simulink model "stepper_motor_driver_model"  (R2012b)
settings: Solver=ode45  StartTime=0.0  StopTime=10.0  RelTol=1e-3
libraries: elec_lib x21, fl_lib x10, nesl_utility x6
settings Model: Creator=Computer  LastModifiedBy=Computer

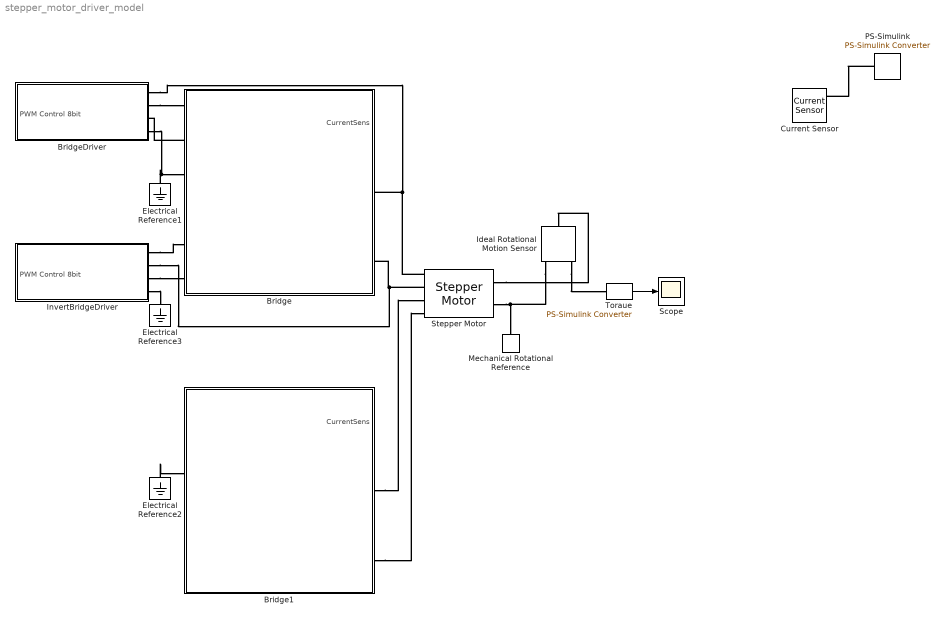
== system stepper_motor_driver_model ==
  Bridge : Subsystem
  Bridge1 : Subsystem
  BridgeDriver : Subsystem
  Current Sensor : fl_lib/Electrical/Electrical Sensors/Current Sensor  i1_Log=off  v1_Log=off  LocalVarNames=|i1|v1  LocalVarDescs=|i1|v1  LocalVarLogging=[0 0]
  Electrical Reference1 : fl_lib/Electrical/Electrical Elements/Electrical Reference  i_Log=off  LocalVarNames=|v1  LocalVarDescs=|v1  LocalVarLogging=[]
  Electrical Reference2 : fl_lib/Electrical/Electrical Elements/Electrical Reference  i_Log=off  LocalVarNames=|v1  LocalVarDescs=|v1  LocalVarLogging=[]
  Electrical Reference3 : fl_lib/Electrical/Electrical Elements/Electrical Reference  i_Log=off  LocalVarNames=|v1  LocalVarDescs=|v1  LocalVarLogging=[]
  Ideal Rotational Motion Sensor : fl_lib/Mechanical/Mechanical Sensors/Ideal Rotational Motion Sensor  offset=0 rad  w_Log=off  t_Log=off  phi_Log=off  LocalVarNames=|w|t|phi  LocalVarDescs=|w|t|phi  LocalVarLogging=[]
  InvertBridgeDriver : Subsystem
  Mechanical Rotational Reference : fl_lib/Mechanical/Rotational Elements/Mechanical Rotational Reference  t_Log=off  LocalVarNames=|t  LocalVarDescs=|t  LocalVarLogging=0
  PS-Simulink : nesl_utility/PS-Simulink Converter  PhysicalDomain=network_engine_domain  LeftPortType=input  RightPortType=output  SubClassName=ps_output  PseudoPeriodic=off  Frequencies=[]  Unit=A  AffineConversion=off
  Scope : Scope
  Stepper Motor : elec_lib/Actuators & Drivers/Rotational Actuators/Stepper Motor  Ra=0.55 Ohm  La=0.0015 H  Km=0.19 N*m/A  Rm=Inf Ohm  Step=1.8 deg  J=4.5e-5 kg*m^2  B=8e-4 N*m/(rad/s)  speed0=0 rpm  theta0=0 deg  LocalVarLogging=[]  alpha=[ 0.00393 0.00393 ] 1/K  Tmeas=25 C  thermal_masses=[ 100 100 ] J/K  initial_temperatures=[ 25 25 ] C  rotor_thermal_mass=50 J/K  rotor_initial_temperature=25 C  Rm_percent_rotor=90
  "Toraue " : nesl_utility/PS-Simulink Converter  PhysicalDomain=network_engine_domain  LeftPortType=input  RightPortType=output  SubClassName=ps_output  PseudoPeriodic=off  Frequencies=[]  Unit=N*m  AffineConversion=off
  wires:
  "Toraue "/1 -> Scope/1
  connections:
  Stepper Motor/RConn2 -- Ideal Rotational Motion Sensor/RConn1 -- Mechanical Rotational Reference/LConn1
  Ideal Rotational Motion Sensor/RConn3 -- "Toraue "/LConn1
  Stepper Motor/RConn1 -- Ideal Rotational Motion Sensor/LConn1
  PS-Simulink/LConn1 -- Current Sensor/RConn1
  Stepper Motor/LConn2 -- InvertBridgeDriver/RConn2 -- Bridge/RConn2
  Stepper Motor/LConn1 -- BridgeDriver/RConn1 -- Bridge/RConn1
  Bridge1/RConn1 -- Stepper Motor/LConn3
  Bridge1/RConn2 -- Stepper Motor/LConn4
  Electrical Reference1/LConn1 -- BridgeDriver/RConn4 -- Bridge/LConn3
  Electrical Reference2/LConn1 -- Bridge1/LConn3
  Bridge/LConn2 -- BridgeDriver/RConn3
  BridgeDriver/RConn2 -- Bridge/LConn1
  InvertBridgeDriver/RConn4 -- Electrical Reference3/LConn1
  InvertBridgeDriver/RConn3 -- Bridge/LConn6
  InvertBridgeDriver/RConn1 -- Bridge/LConn5

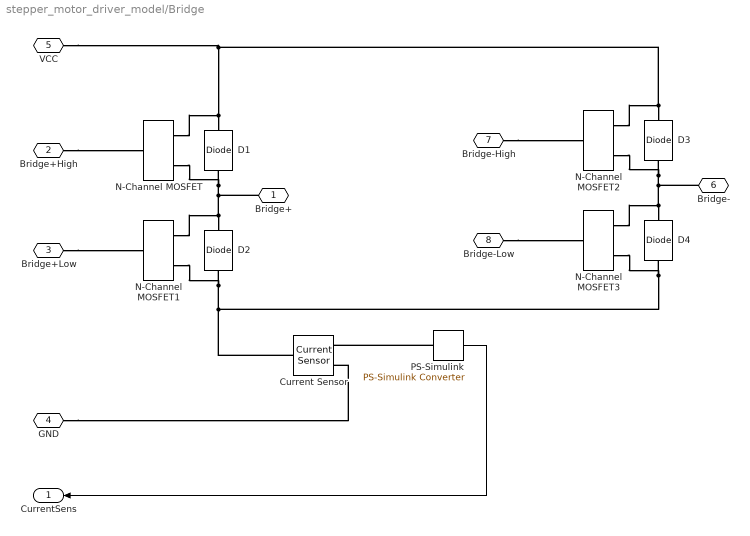
== system stepper_motor_driver_model/Bridge ==
  Current Sensor : fl_lib/Electrical/Electrical Sensors/Current Sensor  i1_Log=off  v1_Log=off  LocalVarNames=|i1|v1  LocalVarDescs=|i1|v1  LocalVarLogging=[0 0]
  D{1..4} (4 alike) : elec_lib/Semiconductor Devices/Diode  ModelType=3  Vf=0.6 V  Ron=0.3 Ohm  Goff=1e-8 S  Rz=0.3 Ohm  Vz=50 V  C_PWL=5 pF  prmExp=1  I12=[ 0.25 5 ] A  V12=[ 0.7 0.8 ] V  I1=0.07 A  V1=0.7 V  RS=0.01 Ohm  IS=1e-14 A  Tmeas=25 C  ec=1  BV=Inf V  C_param=1  CJ0=100 pF  VJ=1 V  Mgrad=0.5  Vvec=[ 0.1 10 100 ] V  Cvec=[ 3.5 1 0.4 ] pF  FC=0.5  Q_param=1  Irrm=-7.15 A  iF=4 A  didt=-750 A/us  trr=115 ns  TT=50 ns  tau=100 ns  T_param=1  IS_T2=1.25e-7 A  I1_T2=0.245 A  V1_T2=0.5 V  Tmeas2=125 C  EG_param=1  EG=1.11 eV  XTI_param=1  XTI=3  dBVdT=0 V/K  Tdevice=25 C  LocalVarLogging=[]  Rth=[ 0 10 ] K/W  thermal_mass_parameterization=1  thermal_mass=[ 0 1 ] J/K  thermal_time_constant=[ 0 10 ] s  thermal_mass_initial_temperatures=[ 25 25 ] C
  N-Channel MOSFET{,1..3} (4 alike) : elec_lib/Semiconductor Devices/N-Channel MOSFET  parameterization=1  prmDatasheet=1  prmEquCoeff=1  Beta=5 A/V^2  Rds=0.025 Ohm  Id=6 A  Vgs=10 V  Vth=1.7 V  lam=0 1/V  Tmeas=25 C  RS=1e-4 Ohm  RD=0.01 Ohm  C_param=1  C_GS=270 pF  C_GD=80 pF  C_iss=350 pF  C_rss=80 pF  dVth_dT=-6 mV/K  Rds_T2=0.037 Ohm  Tmeas2=125 C  BEXDatasheet=-1.5  BEXEquCoeff=-1.5  TdeviceDatasheet=25 C  TdeviceEquCoeff=25 C  LocalVarLogging=[]  Rth=[ 0 10 ] K/W  thermal_mass_parameterization=1  thermal_mass=[ 0 1 ] J/K  thermal_time_constant=[ 0 10 ] s  thermal_mass_initial_temperatures=[ 25 25 ] C
  PS-Simulink : nesl_utility/PS-Simulink Converter  PhysicalDomain=network_engine_domain  LeftPortType=input  RightPortType=output  SubClassName=ps_output  PseudoPeriodic=off  Frequencies=[]  Unit=A  AffineConversion=off
  Bridge+ : PMIOPort  Port=1  Side=Right
  Bridge+High : PMIOPort  Port=2  Side=Left
  Bridge+Low : PMIOPort  Port=3  Side=Left
  "GND " : PMIOPort  Port=4  Side=Left
  VCC : PMIOPort  Port=5  Side=Left
  Bridge- : PMIOPort  Port=6  Side=Right
  Bridge-High : PMIOPort  Port=7  Side=Left
  Bridge-Low : PMIOPort  Port=8  Side=Left
  CurrentSens : Outport
  wires:
  PS-Simulink/1 -> CurrentSens/1
  connections:
  N-Channel MOSFET1/RConn1 -- Bridge+/RConn1 -- N-Channel MOSFET/RConn2 -- D1/LConn1 -- D2/RConn1
  D4/LConn1 -- N-Channel MOSFET1/RConn2 -- D2/LConn1 -- Current Sensor/LConn1 -- N-Channel MOSFET3/RConn2
  N-Channel MOSFET2/RConn1 -- D1/RConn1 -- N-Channel MOSFET/RConn1 -- VCC/RConn1 -- D3/RConn1
  Bridge+High/RConn1 -- N-Channel MOSFET/LConn1
  Bridge+Low/RConn1 -- N-Channel MOSFET1/LConn1
  PS-Simulink/LConn1 -- Current Sensor/RConn1
  "GND "/RConn1 -- Current Sensor/RConn2
  N-Channel MOSFET3/RConn1 -- Bridge-/RConn1 -- N-Channel MOSFET2/RConn2 -- D3/LConn1 -- D4/RConn1
  Bridge-High/RConn1 -- N-Channel MOSFET2/LConn1
  Bridge-Low/RConn1 -- N-Channel MOSFET3/LConn1

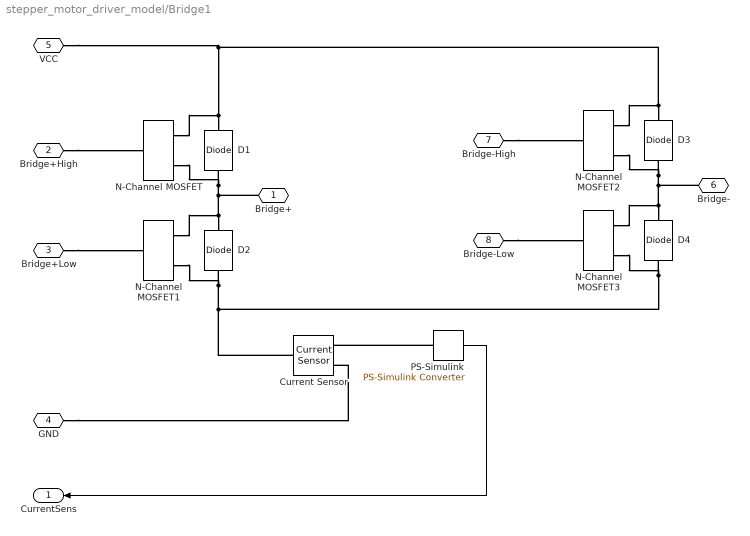
== system stepper_motor_driver_model/Bridge1 ==
  Current Sensor : fl_lib/Electrical/Electrical Sensors/Current Sensor  i1_Log=off  v1_Log=off  LocalVarNames=|i1|v1  LocalVarDescs=|i1|v1  LocalVarLogging=[0 0]
  D{1..4} (4 alike) : elec_lib/Semiconductor Devices/Diode  ModelType=3  Vf=0.6 V  Ron=0.3 Ohm  Goff=1e-8 S  Rz=0.3 Ohm  Vz=50 V  C_PWL=5 pF  prmExp=1  I12=[ 0.25 5 ] A  V12=[ 0.7 0.8 ] V  I1=0.07 A  V1=0.7 V  RS=0.01 Ohm  IS=1e-14 A  Tmeas=25 C  ec=1  BV=Inf V  C_param=1  CJ0=100 pF  VJ=1 V  Mgrad=0.5  Vvec=[ 0.1 10 100 ] V  Cvec=[ 3.5 1 0.4 ] pF  FC=0.5  Q_param=1  Irrm=-7.15 A  iF=4 A  didt=-750 A/us  trr=115 ns  TT=50 ns  tau=100 ns  T_param=1  IS_T2=1.25e-7 A  I1_T2=0.245 A  V1_T2=0.5 V  Tmeas2=125 C  EG_param=1  EG=1.11 eV  XTI_param=1  XTI=3  dBVdT=0 V/K  Tdevice=25 C  LocalVarLogging=[]  Rth=[ 0 10 ] K/W  thermal_mass_parameterization=1  thermal_mass=[ 0 1 ] J/K  thermal_time_constant=[ 0 10 ] s  thermal_mass_initial_temperatures=[ 25 25 ] C
  N-Channel MOSFET{,1..3} (4 alike) : elec_lib/Semiconductor Devices/N-Channel MOSFET  parameterization=1  prmDatasheet=1  prmEquCoeff=1  Beta=5 A/V^2  Rds=0.025 Ohm  Id=6 A  Vgs=10 V  Vth=1.7 V  lam=0 1/V  Tmeas=25 C  RS=1e-4 Ohm  RD=0.01 Ohm  C_param=1  C_GS=270 pF  C_GD=80 pF  C_iss=350 pF  C_rss=80 pF  dVth_dT=-6 mV/K  Rds_T2=0.037 Ohm  Tmeas2=125 C  BEXDatasheet=-1.5  BEXEquCoeff=-1.5  TdeviceDatasheet=25 C  TdeviceEquCoeff=25 C  LocalVarLogging=[]  Rth=[ 0 10 ] K/W  thermal_mass_parameterization=1  thermal_mass=[ 0 1 ] J/K  thermal_time_constant=[ 0 10 ] s  thermal_mass_initial_temperatures=[ 25 25 ] C
  PS-Simulink : nesl_utility/PS-Simulink Converter  PhysicalDomain=network_engine_domain  LeftPortType=input  RightPortType=output  SubClassName=ps_output  PseudoPeriodic=off  Frequencies=[]  Unit=A  AffineConversion=off
  Bridge+ : PMIOPort  Port=1  Side=Right
  Bridge+High : PMIOPort  Port=2  Side=Left
  Bridge+Low : PMIOPort  Port=3  Side=Left
  "GND " : PMIOPort  Port=4  Side=Left
  VCC : PMIOPort  Port=5  Side=Left
  Bridge- : PMIOPort  Port=6  Side=Right
  Bridge-High : PMIOPort  Port=7  Side=Left
  Bridge-Low : PMIOPort  Port=8  Side=Left
  CurrentSens : Outport
  wires:
  PS-Simulink/1 -> CurrentSens/1
  connections:
  N-Channel MOSFET/RConn2 -- D1/LConn1 -- D2/RConn1 -- N-Channel MOSFET1/RConn1 -- Bridge+/RConn1
  N-Channel MOSFET1/RConn2 -- D2/LConn1 -- Current Sensor/LConn1 -- N-Channel MOSFET3/RConn2 -- D4/LConn1
  D1/RConn1 -- N-Channel MOSFET/RConn1 -- VCC/RConn1 -- D3/RConn1 -- N-Channel MOSFET2/RConn1
  Bridge+High/RConn1 -- N-Channel MOSFET/LConn1
  Bridge+Low/RConn1 -- N-Channel MOSFET1/LConn1
  PS-Simulink/LConn1 -- Current Sensor/RConn1
  "GND "/RConn1 -- Current Sensor/RConn2
  Bridge-/RConn1 -- N-Channel MOSFET2/RConn2 -- D3/LConn1 -- D4/RConn1 -- N-Channel MOSFET3/RConn1
  Bridge-High/RConn1 -- N-Channel MOSFET2/LConn1
  Bridge-Low/RConn1 -- N-Channel MOSFET3/LConn1

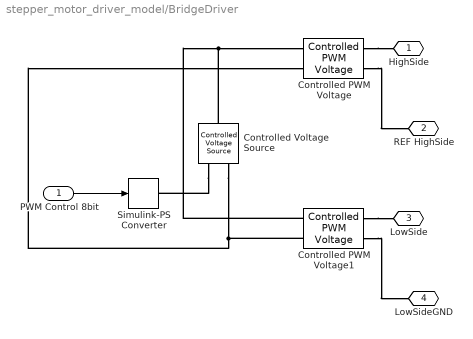
== system stepper_motor_driver_model/BridgeDriver ==
  PWM Control 8bit : Inport
  Controlled PWM Voltage : elec_lib/Actuators & Drivers/Drivers/Controlled PWM Voltage  F=150 kHz  TD=0 s  pulse_width_offset=0 s  Vmin=0 V  Vmax=255 V  Vm=10 V  pwm_or_av=1  event_type=1  sample_time=1e-6 s  LocalVarLogging=[]
  Controlled PWM Voltage1 : elec_lib/Actuators & Drivers/Drivers/Controlled PWM Voltage  F=150 kHz  TD=0 s  pulse_width_offset=0 s  Vmin=0 V  Vmax=255 V  Vm=10 V  pwm_or_av=1  event_type=1  sample_time=1e-6 s  LocalVarLogging=[]
  Controlled Voltage Source : fl_lib/Electrical/Electrical Sources/Controlled Voltage Source  i_Log=off  v_Log=off  LocalVarNames=|current|voltage|power  LocalVarDescs=|Current (A)|Voltage (V)|Power (W)  LocalVarLogging=[0 0 0]
  Simulink-PS Converter : nesl_utility/Simulink-PS Converter  PhysicalDomain=network_engine_domain  LeftPortType=input  RightPortType=output  SubClassName=ps_input  PseudoPeriodic=off  Frequencies=[]  NoiseDistribution=none  NoiseParameters=[]  Unit=V  AffineConversion=off  InputFilterTimeConstant=.001  UdotUserProvided=0  SimscapeFilterOrder=1  InputFiltering=off
  HighSide : PMIOPort  Port=1  Side=Right
  REF HighSide : PMIOPort  Port=2  Side=Right
  LowSide : PMIOPort  Port=3  Side=Right
  LowSideGND : PMIOPort  Port=4  Side=Right
  wires:
  PWM Control 8bit/1 -> Simulink-PS Converter/1
  connections:
  Controlled PWM Voltage/RConn1 -- HighSide/RConn1
  Controlled PWM Voltage/RConn2 -- REF HighSide/RConn1
  Controlled PWM Voltage1/RConn2 -- LowSideGND/RConn1
  Controlled PWM Voltage1/RConn1 -- LowSide/RConn1
  Controlled Voltage Source/RConn1 -- Simulink-PS Converter/RConn1
  Controlled Voltage Source/LConn1 -- Controlled PWM Voltage/LConn1 -- Controlled PWM Voltage1/LConn1
  Controlled Voltage Source/RConn2 -- Controlled PWM Voltage1/LConn2 -- Controlled PWM Voltage/LConn2

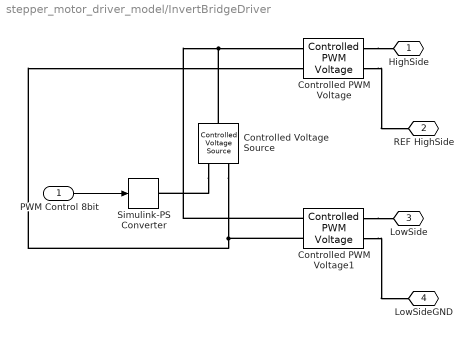
== system stepper_motor_driver_model/InvertBridgeDriver ==
  PWM Control 8bit : Inport
  Controlled PWM Voltage : elec_lib/Actuators & Drivers/Drivers/Controlled PWM Voltage  F=150 kHz  TD=0 s  pulse_width_offset=0 s  Vmin=0 V  Vmax=-255 V  Vm=10 V  pwm_or_av=1  event_type=1  sample_time=1e-6 s  LocalVarLogging=[]
  Controlled PWM Voltage1 : elec_lib/Actuators & Drivers/Drivers/Controlled PWM Voltage  F=150 kHz  TD=0 s  pulse_width_offset=0 s  Vmin=0 V  Vmax=-255 V  Vm=10 V  pwm_or_av=1  event_type=1  sample_time=1e-6 s  LocalVarLogging=[]
  Controlled Voltage Source : fl_lib/Electrical/Electrical Sources/Controlled Voltage Source  i_Log=off  v_Log=off  LocalVarNames=|current|voltage|power  LocalVarDescs=|Current (A)|Voltage (V)|Power (W)  LocalVarLogging=[0 0 0]
  Simulink-PS Converter : nesl_utility/Simulink-PS Converter  PhysicalDomain=network_engine_domain  LeftPortType=input  RightPortType=output  SubClassName=ps_input  PseudoPeriodic=off  Frequencies=[]  NoiseDistribution=none  NoiseParameters=[]  Unit=V  AffineConversion=off  InputFilterTimeConstant=.001  UdotUserProvided=0  SimscapeFilterOrder=1  InputFiltering=off
  HighSide : PMIOPort  Port=1  Side=Right
  REF HighSide : PMIOPort  Port=2  Side=Right
  LowSide : PMIOPort  Port=3  Side=Right
  LowSideGND : PMIOPort  Port=4  Side=Right
  wires:
  PWM Control 8bit/1 -> Simulink-PS Converter/1
  connections:
  Controlled PWM Voltage/RConn1 -- HighSide/RConn1
  Controlled PWM Voltage/RConn2 -- REF HighSide/RConn1
  Controlled PWM Voltage1/RConn2 -- LowSideGND/RConn1
  Controlled PWM Voltage1/RConn1 -- LowSide/RConn1
  Controlled Voltage Source/RConn1 -- Simulink-PS Converter/RConn1
  Controlled PWM Voltage1/LConn1 -- Controlled Voltage Source/LConn1 -- Controlled PWM Voltage/LConn1
  Controlled Voltage Source/RConn2 -- Controlled PWM Voltage/LConn2 -- Controlled PWM Voltage1/LConn2
